simulink model "IDMF_datagenerator"  (R2022a)
settings: Solver=VariableStepAuto  StartTime=0.0  StopTime=30  FixedStep=0.05  RelTol=1e-3
PostLoadFcn:
  | %Add subfolders to path
  | addpath('virtualworld');
InitFcn:
  | startScript;
values from neighbouring files (symbols this model uses):
  angularVelocity = [0 0 -0.01]    [startScript.m]
  angularVelocityforLanding = [0 0 0]    [startScript.m]
  dronestartlocation = [-1.5 0 4]    [startScript.m]
  Dstar = -0.5    [startScript.m]
  finalHoverHeight = 2.5    [startScript.m]
  helipadLocation = [14 0.6 5]    [startScript.m]
  linearVelocity = [5 0.05 1]    [startScript.m]
  linearVelocityforHover = [0.65 0.05 0.3]    [startScript.m]
  windAVelocity = [0 0.1 0.1]    [startScript.m]
  windLVelocity = [0.1 0 0.3]    [startScript.m]
undefined symbols (not defined in the file or in its folder): fspecial, gcbh, Kanade, Lucas, Rec, SDTV, vrmfunc
libraries: visiontextngfix x11, visionconversions x9, visionanalysis x8, vrlib x7, slpidlib x3, sharedtransform x2, simulink x1
(part 1 of 3)
settings Model: Creator=91967  LastModifiedBy=sshoo
settings SolverCC: AlgebraicLoopSolver=TrustRegion
settings DebuggingCC: UnconnectedInputMsg=warning  UnconnectedOutputMsg=warning  UnconnectedLineMsg=warning  SFMachineParentedDataDiag=warning
settings SFSimCC: MATLABDynamicMemAllocThreshold=4000
settings RTWCC: DLArmComputeVersion=19.05

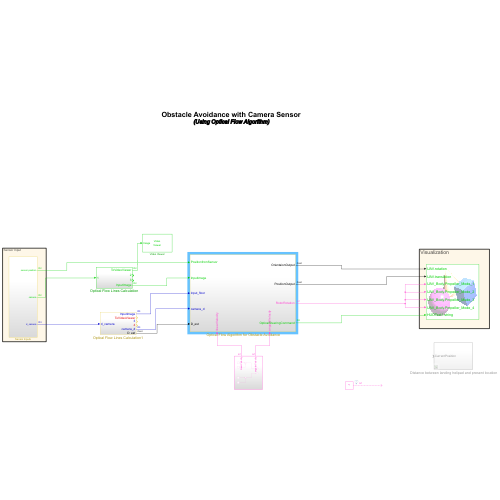
[thumbnail: Simulink's stored preview of the top-level diagram]
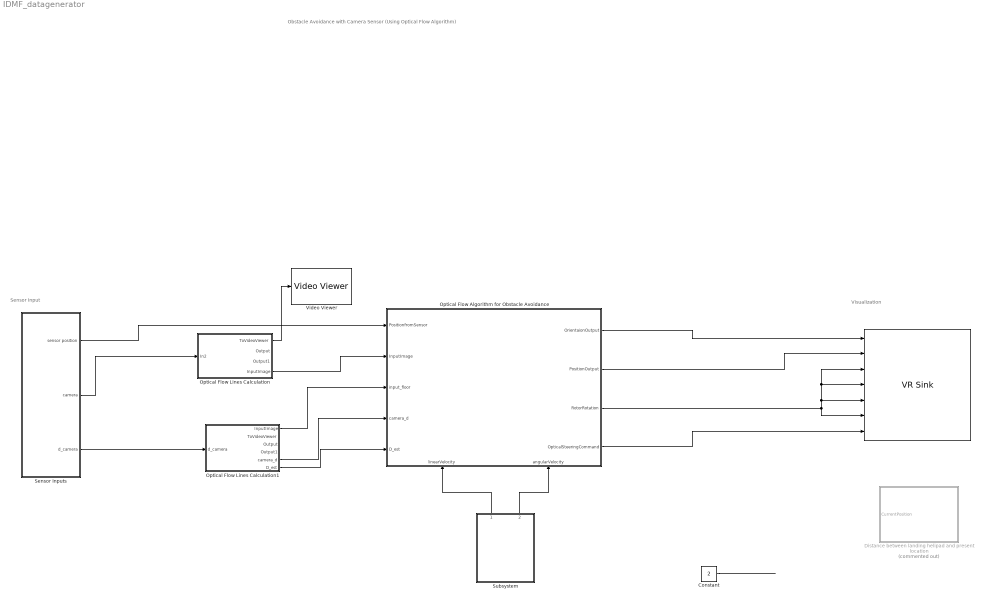
== system IDMF_datagenerator ==
  note: Sensor Input
  note: Obstacle Avoidance with Camera Sensor
      | (Using Optical Flow Algorithm)
  note: Visualization
  "    " : vrlib/VR Sink  InstantiateOnLoad=on  SampleTime=0.04  ViewEnable=on  RemoteChange=off  RemoteView=off  FieldsWritten=UAV.rotation.4.1.1.double#UAV.translation.3.1.1.double#UAV_Body.Propeller_Mode_1.1.1.1.double#UAV_Body.Propeller_Mode_2.1.1.1.double#UAV_Body.Propeller_Mode_3.1.1.1.double#UAV_Body.Propeller_Mode_4.1.1.1.double#HUDText1.string.1.-1.1.char  WorldFileName=slv3.x3d  WorldDescription=Obstacle Avoidance with Camera Sensor (Using Optical Flow Algorithm)  AutoView=off  VideoDimensions=[]  AllowVariableSize=off
  " Distance between landing helipad and present location" : Subsystem  Commented=on
  " Optical Flow Algorithm for Obstacle Avoidance" : Subsystem
      settings: PortSchema="{\"entries\":[{\"content\":{\"sides\":[{\"content\":{\"connectorIds\":[\"In1\",\"In2\",\"In3\",\"In4\",\"In5\"]},\"type\":\"ConnectorPlacement.EquallySpacedRectSide\",\"uuid\":\"626d938a-dc4f-460f-bc0f-94d4819770df\"},{\"content\":{\"connectorIds\":[\"Out1\",\"Out2\",\"Out3\",\"Out4\"],\"side\":\"RIGHT\"},\"type\":\"ConnectorPlacement.EquallySpacedRectSide\",\"uuid\":\"f8576f54-f0f3-45bb-99e7-76b9dd7ef3ed\"},{\"content\":{\"connectorIds\":[],\"side\":\"TOP\"},\"type\":\"ConnectorPlacement.EquallySpacedRectSide\",\"uuid\":\"339010c6-3d09-402d-955a-c6f9b5dbd0bd\"},{\"content\":{\"connectorIds\":[\"In6\",\"In7\"],\"side\":\"BOTTOM\"},\"type\":\"ConnectorPlacement.EquallySpacedRectSide\",\"uuid\":\"67e63212-85fa-4929-bde2-eaa65e03c106\"}]},\"type\":\"ConnectorPlacement.EquallySpacedConnector\",\"uuid\":\"635d6afa-5e1d-48cf-844f-d5ce6ee259d5\"}],\"packageUris\":[\"http://schema.mathworks.com/mf0/Connector/R2020b\"],\"version\":\"1.0\"}"
  Constant : Constant  Value=2
  Optical Flow Lines Calculation : Subsystem
  Optical Flow Lines Calculation1 : Subsystem
  Sensor Inputs : Subsystem
  Subsystem : Subsystem
  Video Viewer : VideoViewer  FigPos=[100 1042 709 500]
  wires:
  Sensor Inputs/1(sensor position) -> " Optical Flow Algorithm for Obstacle Avoidance"/1(PositionfromSensor)
  Sensor Inputs/2(camera) -> Optical Flow Lines Calculation/1(In2)
  " Optical Flow Algorithm for Obstacle Avoidance"/3(RotorRotation) -> "    "/6, "    "/4, "    "/3, "    "/5
  " Optical Flow Algorithm for Obstacle Avoidance"/4(OpticalSteeringCommand) -> "    "/7
  Sensor Inputs/3(d_camera) -> Optical Flow Lines Calculation1/1(d_camera)
  Optical Flow Lines Calculation1/1(InputImage) -> " Optical Flow Algorithm for Obstacle Avoidance"/3(input_floor)
  Optical Flow Lines Calculation/4(InputImage) -> " Optical Flow Algorithm for Obstacle Avoidance"/2(InputImage)
  Optical Flow Lines Calculation1/6(D_est) -> " Optical Flow Algorithm for Obstacle Avoidance"/5(D_est)
  Optical Flow Lines Calculation1/5(camera_d) -> " Optical Flow Algorithm for Obstacle Avoidance"/4(camera_d)
  " Optical Flow Algorithm for Obstacle Avoidance"/1(OrientaionOutput) -> "    "/1
  " Optical Flow Algorithm for Obstacle Avoidance"/2(PositionOutput) -> "    "/2
  Subsystem/1(linearVelocity) -> " Optical Flow Algorithm for Obstacle Avoidance"/6(linearVelocity)
  Subsystem/2(angularVelocity) -> " Optical Flow Algorithm for Obstacle Avoidance"/7(angularVelocity)
  Constant/1 -> ?
  Optical Flow Lines Calculation/1(ToVideoViewer) -> Video Viewer/1

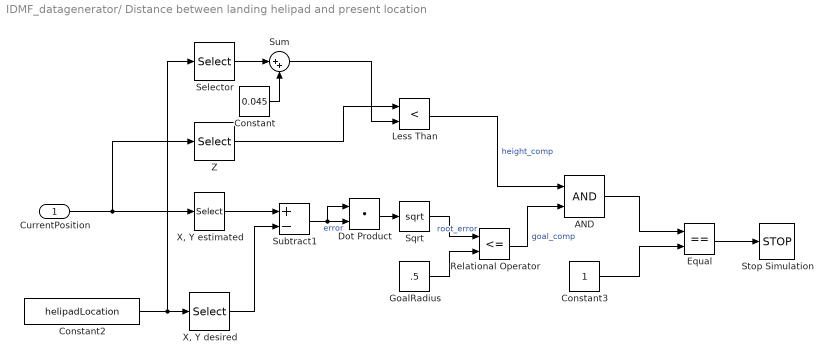
== system IDMF_datagenerator/ Distance between landing helipad and present location ==
  CurrentPosition : Inport
  AND : Logic  IconShape=distinctive  AllPortsSameDT=off  OutDataTypeStr=boolean
  Constant : Constant  Value=0.045
  Constant2 : Constant  Value=helipadLocation
  Constant3 : Constant
  Dot Product : DotProduct  OutDataTypeStr=Inherit: Inherit via internal rule
  Equal : RelationalOperator  Operator===  OutDataTypeStr=boolean  RndMeth=Simplest  InputSameDT=off
  GoalRadius : Constant  Value=.5
  Less Than : RelationalOperator  Operator=<  OutDataTypeStr=boolean  RndMeth=Simplest  InputSameDT=off
  Relational Operator : RelationalOperator  Operator=<=  OutDataTypeStr=boolean  RndMeth=Simplest  InputSameDT=off
  Selector : Selector  InputPortWidth=3  IndexOptions=Index vector (dialog)  Indices=[2]  OutputSizes=1
  Sqrt : Sqrt
  Stop Simulation : Stop
  Subtract1 : Sum  Inputs=+-
  Sum : Sum  Inputs=|++
  "X, Y desired" : Selector  InputPortWidth=3  IndexOptions=Index vector (dialog)  Indices=[1 3]  OutputSizes=1
  "X, Y estimated" : Selector  InputPortWidth=3  IndexOptions=Index vector (dialog)  Indices=[1 3]  OutputSizes=1
  Z : Selector  InputPortWidth=3  IndexOptions=Index vector (dialog)  Indices=[2]  OutputSizes=1
  wires:
  GoalRadius/1 -> Relational Operator/2
  Subtract1/1 -> Dot Product/1, Dot Product/2  "error"
  Dot Product/1 -> Sqrt/1
  Sqrt/1 -> Relational Operator/1  "root_error"
  "X, Y estimated"/1 -> Subtract1/1
  CurrentPosition/1 -> Z/1, "X, Y estimated"/1
  "X, Y desired"/1 -> Subtract1/2
  Constant3/1 -> Equal/2
  Equal/1 -> Stop Simulation/1
  Constant2/1 -> Selector/1, "X, Y desired"/1
  AND/1 -> Equal/1
  Relational Operator/1 -> AND/2  "goal_comp"
  Z/1 -> Less Than/1
  Less Than/1 -> AND/1  "height_comp"
  Selector/1 -> Sum/1
  Constant/1 -> Sum/2
  Sum/1 -> Less Than/2

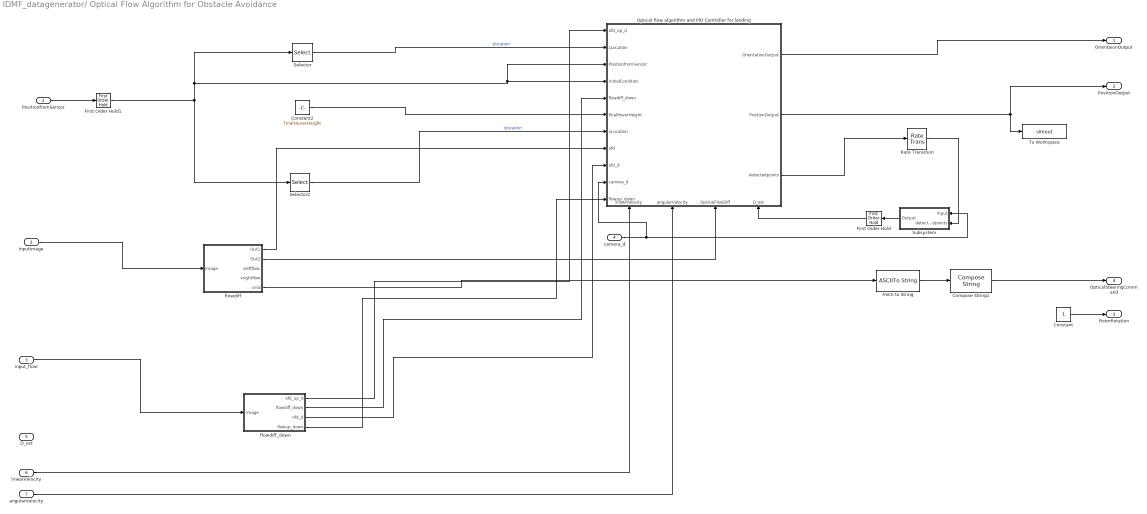
== system IDMF_datagenerator/ Optical Flow Algorithm for Obstacle Avoidance ==
  PositionfromSensor : Inport  OutDataTypeStr=double
  InputImage : Inport  Port=2
  input_floor : Inport  Port=3
  camera_d : Inport  Port=4
  D_est : Inport  Port=5
  linearVelocity : Inport  Port=6
  angularVelocity : Inport  Port=7
  ASCII to String : ASCIIToString
  Compose String1 : ComposeString  Format="\"%s\""
  Constant : Constant
  Constant2 : Constant  Value=finalHoverHeight
  First Order Hold : FirstOrderHold  ErrorTolerance=0  AllowContinuousInput=on
  First Order Hold1 : FirstOrderHold  ErrorTolerance=inf
  Optical flow algorithm and PID Controller for landing : Stateflow chart  TreatAsAtomicUnit=on
      settings: PortSchema="{\"entries\":[{\"content\":{\"sides\":[{\"content\":{\"connectorIds\":[\"In5\",\"In6\",\"In7\",\"In8\",\"In9\",\"In10\",\"In11\",\"In13\",\"In14\",\"In12\",\"In15\"]},\"type\":\"ConnectorPlacement.EquallySpacedRectSide\",\"uuid\":\"e0417acb-7520-44a1-81fe-3cf9a64aaaa4\"},{\"content\":{\"connectorIds\":[\"Out1\",\"Out2\",\"Out3\"],\"side\":\"RIGHT\"},\"type\":\"ConnectorPlacement.EquallySpacedRectSide\",\"uuid\":\"44842af9-d70e-40e5-b27b-20e9bdb5de5c\"},{\"content\":{\"connectorIds\":[],\"side\":\"TOP\"},\"type\":\"ConnectorPlacement.EquallySpacedRectSide\",\"uuid\":\"27a245c1-5cf2-418b-a56f-6add92dc71be\"},{\"content\":{\"connectorIds\":[\"In1\",\"In2\",\"In3\",\"In4\"],\"side\":\"BOTTOM\"},\"type\":\"ConnectorPlacement.EquallySpacedRectSide\",\"uuid\":\"f0be2f5a-19b7-4698-85a9-69c72a6e07e4\"}]},\"type\":\"ConnectorPlacement.EquallySpacedConnector\",\"uuid\":\"6007b39c-018d-48d6-ae79-01dba3bf1617\"}],\"packageUris\":[\"http://schema.mathworks.com/mf0/Connector/R2020b\"],\"version\":\"1.0\"}"
  Rate Transition : RateTransition  OutPortSampleTime=0.1
  Selector : Selector  InputPortWidth=3  IndexOptions=Index vector (dialog)  Indices=[2]  OutputSizes=1
  Selector2 : Selector  InputPortWidth=3  IndexOptions=Index vector (dialog)  Indices=[1]  OutputSizes=1
  Subsystem : Subsystem
  To Workspace : ToWorkspace  VariableName=simout  SaveFormat=Timeseries  SampleTime=-1
  flowdiff : Subsystem
  flowdiff_down : Subsystem
  OrientaionOutput : Outport
  PositionOutput : Outport  Port=2
  RotorRotation : Outport  Port=3
  OpticalSteeringCommand : Outport  Port=4
  wires:
  Optical flow algorithm and PID Controller for landing/2(PositionOutput) -> PositionOutput/1, To Workspace/1
  Optical flow algorithm and PID Controller for landing/1(OrientationOutput) -> OrientaionOutput/1
  ASCII to String/1 -> Compose String1/1
  Compose String1/1 -> OpticalSteeringCommand/1
  Constant/1 -> RotorRotation/1
  PositionfromSensor/1 -> First Order Hold1/1
  Selector/1 -> Optical flow algorithm and PID Controller for landing/6(zLocation)  "zlocation"
  Constant2/1 -> Optical flow algorithm and PID Controller for landing/10(finalHoverHeight)
  Selector2/1 -> Optical flow algorithm and PID Controller for landing/11(xLocation)  "xlocation"
  camera_d/1 -> Optical flow algorithm and PID Controller for landing/12(camera_d), Subsystem/1(Input)
  Optical flow algorithm and PID Controller for landing/3(detectedpoints) -> Rate Transition/1
  Rate Transition/1 -> Subsystem/2(detectedpoints)
  First Order Hold/1 -> Optical flow algorithm and PID Controller for landing/4(D_est)
  Subsystem/1(Output) -> First Order Hold/1
  input_floor/1 -> flowdiff_down/1(image)
  flowdiff_down/1(ofd_up_d) -> Optical flow algorithm and PID Controller for landing/5(ofd_up_d)
  flowdiff_down/2(flowdiff_down) -> Optical flow algorithm and PID Controller for landing/9(flowdiff_down)
  flowdiff_down/3(ofd_d) -> Optical flow algorithm and PID Controller for landing/14(ofd_d)
  flowdiff_down/4(flowup_down) -> Optical flow algorithm and PID Controller for landing/15(flowup_down)
  InputImage/1 -> flowdiff/1(image)
  flowdiff/1(Out1) -> Optical flow algorithm and PID Controller for landing/13(ofd)
  flowdiff/2(Out2) -> Optical flow algorithm and PID Controller for landing/3(OpticalFlowDiff)
  flowdiff/5(cmd) -> ASCII to String/1
  linearVelocity/1 -> Optical flow algorithm and PID Controller for landing/1(linearVelocity)
  angularVelocity/1 -> Optical flow algorithm and PID Controller for landing/2(angularVelocity)
  First Order Hold1/1 -> Selector/1, Optical flow algorithm and PID Controller for landing/7(PositionfromSensor), Optical flow algorithm and PID Controller for landing/8(InitialCondition), Selector2/1

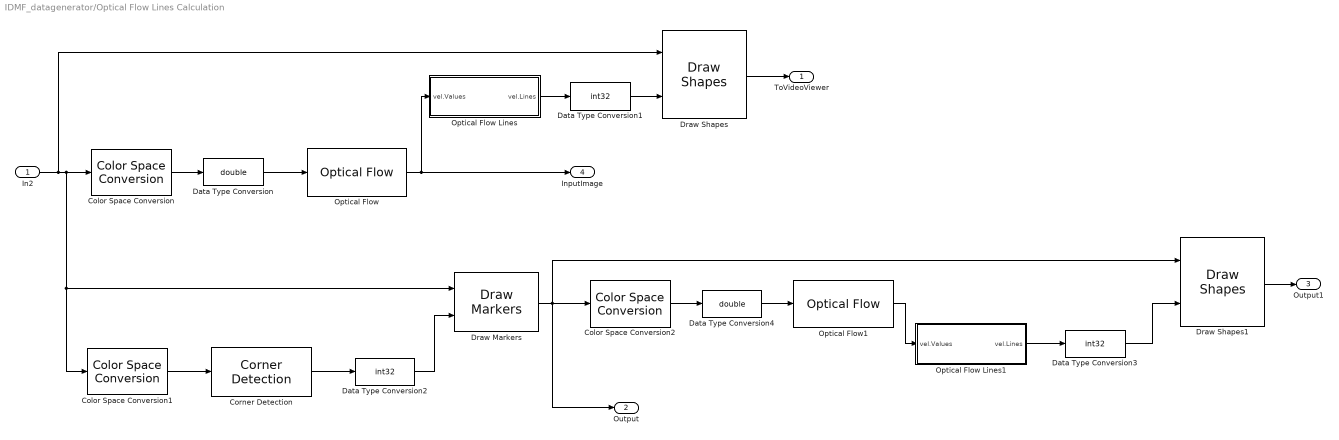
== system IDMF_datagenerator/Optical Flow Lines Calculation ==
  In2 : Inport
  Color Space Conversion : visionconversions/Color Space  Conversion  conversion=Obsolete  conversionActive=R'G'B' to intensity  wp_str=D65  rec=Rec. 601 (SDTV)  sys=1125/60/2:1  imagePorts=One multidimensional signal
  Color Space Conversion1 : visionconversions/Color Space  Conversion  conversion=Obsolete  conversionActive=R'G'B' to intensity  wp_str=D65  rec=Rec. 601 (SDTV)  sys=1125/60/2:1  imagePorts=One multidimensional signal
  Color Space Conversion2 : visionconversions/Color Space  Conversion  conversion=Obsolete  conversionActive=R'G'B' to intensity  wp_str=D65  rec=Rec. 601 (SDTV)  sys=1125/60/2:1  imagePorts=One multidimensional signal
  Corner Detection : visionanalysis/Corner Detection  method=Local intensity comparison (Rosen & Drummond)  factor=0.04  filter=fspecial('gaussian', [1 5], 1.5)  thrInten=0.1  thrAngle=112.5  output=Obsolete9b  outputInUse=Corner location  maxNum=50  thrMetric=0.005  neighborSize=[11 11]  isOutVarDim=on  roundingMode=Floor  overflowMode=off  firstCoeffMode=Specify word length  firstCoeffWordLength=16  firstCoeffFracLength=16  prodOutputMode=Binary point scaling  prodOutputWordLength=32  prodOutputFracLength=0  accumMode=Binary point scaling  accumWordLength=32  accumFracLength=0  memoryMode=Binary point scaling  memoryWordLength=32  memoryFracLength=0
      settings: SourceProductBaseCode=VP
  Data Type Conversion : DataTypeConversion  OutDataTypeStr=double  SaturateOnIntegerOverflow=off  RndMeth=Floor
  Data Type Conversion1 : DataTypeConversion  OutDataTypeStr=int32  SaturateOnIntegerOverflow=off  RndMeth=Floor
  Data Type Conversion2 : DataTypeConversion  OutDataTypeStr=int32  SaturateOnIntegerOverflow=off  RndMeth=Floor
  Data Type Conversion3 : DataTypeConversion  OutDataTypeStr=int32  SaturateOnIntegerOverflow=off  RndMeth=Floor
  Data Type Conversion4 : DataTypeConversion  OutDataTypeStr=double  SaturateOnIntegerOverflow=off  RndMeth=Floor
  Draw Markers : visiontextngfix/Draw Markers  shape=Plus  size=3  fill=off  fillClrSource=Specify via dialog  display=User-specified value  intensity=200  color=[255 0 0]  opacity=0.6  viewport=Entire image  antialiasing=off  inType=Obsolete  imagePorts=One multidimensional signal  roundingMode=Floor  overflowMode=off  memoryMode=Specify word length  memoryWordLength=16  memoryFracLength=15  prodOutputMode=Binary point scaling  prodOutputWordLength=32  prodOutputFracLength=14
      settings: SourceProductBaseCode=VP
  Draw Shapes : visiontextngfix/Draw Shapes  shape=Lines  fill=off  lineWidth=1  fillClrSource=Specify via dialog  display=User-specified value  intensity=200  color=[255 0 0]  opacity=0.6  viewport=Entire image  antialiasing=off  inType=Obsolete  imagePorts=One multidimensional signal  roundingMode=Floor  overflowMode=off  memoryMode=Specify word length  memoryWordLength=16  prodOutputMode=Binary point scaling  prodOutputWordLength=32  prodOutputFracLength=14  memoryFracLength=15
  Draw Shapes1 : visiontextngfix/Draw Shapes  shape=Lines  fill=off  lineWidth=1  fillClrSource=Specify via dialog  display=User-specified value  intensity=200  color=[255 255 0]  opacity=0.6  viewport=Entire image  antialiasing=off  inType=Obsolete  imagePorts=One multidimensional signal  roundingMode=Floor  overflowMode=off  memoryMode=Specify word length  memoryWordLength=16  prodOutputMode=Binary point scaling  prodOutputWordLength=32  prodOutputFracLength=14  memoryFracLength=15
  Optical Flow : visionanalysis/Optical Flow  method=Lucas-Kanade  gradMethod=Derivative of Gaussian  which2img=Current frame and N-th frame back  N=1  lambda=60  numInports=5  sigmaS=1.5  sigmaW=1  discardNormalFlow=off  outputCurrentImage=off  stop_criteria=When maximum number of iterations is reached  maxIter=10  maxAllowAbsDiff=eps  outVelForm=Magnitude-squared  eigTh=0.039  roundingMode=Nearest  overflowMode=on  prodOutputMode=Binary point scaling  prodOutputWordLength=32  prodOutputFracLength=20  outputMode=Binary point scaling  outputWordLength=32  outputFracLength=20
      settings: SourceProductBaseCode=VP
  Optical Flow Lines : Subsystem  mask(Optical Flow Lines){scaleFactor=1}
      mask prompts: scaleFactor "Motion vector gain:"
      mask help: Generates the coordinate points of optical flow lines.
      mask Help: Generates the coordinate points of optical flow lines. Look under its mask to see the implementation details.
  Optical Flow Lines1 : Subsystem  mask(Optical Flow Lines){scaleFactor=1}
      mask prompts: scaleFactor "Motion vector gain:"
      mask help: Generates the coordinate points of optical flow lines.
      mask Help: Generates the coordinate points of optical flow lines. Look under its mask to see the implementation details.
  Optical Flow1 : visionanalysis/Optical Flow  method=Lucas-Kanade  gradMethod=Derivative of Gaussian  which2img=Current frame and N-th frame back  N=1  lambda=1  numInports=3  sigmaS=1.5  sigmaW=1  discardNormalFlow=off  outputCurrentImage=off  stop_criteria=When maximum number of iterations is reached  maxIter=10  maxAllowAbsDiff=eps  outVelForm=Magnitude-squared  eigTh=0.0039  roundingMode=Nearest  overflowMode=on  prodOutputMode=Binary point scaling  prodOutputWordLength=32  prodOutputFracLength=20  outputMode=Binary point scaling  outputWordLength=32  outputFracLength=20
      settings: SourceProductBaseCode=VP
  ToVideoViewer : Outport
  Output : Outport  Port=2
  Output1 : Outport  Port=3
  InputImage : Outport  Port=4
  wires:
  Optical Flow Lines/1(vel.Lines) -> Data Type Conversion1/1
  Data Type Conversion1/1 -> Draw Shapes/2
  Draw Shapes/1 -> ToVideoViewer/1
  Data Type Conversion/1 -> Optical Flow/1
  Color Space Conversion/1 -> Data Type Conversion/1
  Optical Flow Lines1/1(vel.Lines) -> Data Type Conversion3/1
  Data Type Conversion3/1 -> Draw Shapes1/2
  Draw Shapes1/1 -> Output1/1
  Color Space Conversion2/1 -> Data Type Conversion4/1
  Data Type Conversion4/1 -> Optical Flow1/1
  Corner Detection/1 -> Data Type Conversion2/1
  Draw Markers/1 -> Draw Shapes1/1, Output/1, Color Space Conversion2/1
  Data Type Conversion2/1 -> Draw Markers/2
  Color Space Conversion1/1 -> Corner Detection/1
  Optical Flow1/1 -> Optical Flow Lines1/1(vel.Values)
  In2/1 -> Color Space Conversion1/1, Draw Markers/1, Color Space Conversion/1, Draw Shapes/1
  Optical Flow/1 -> Optical Flow Lines/1(vel.Values), InputImage/1

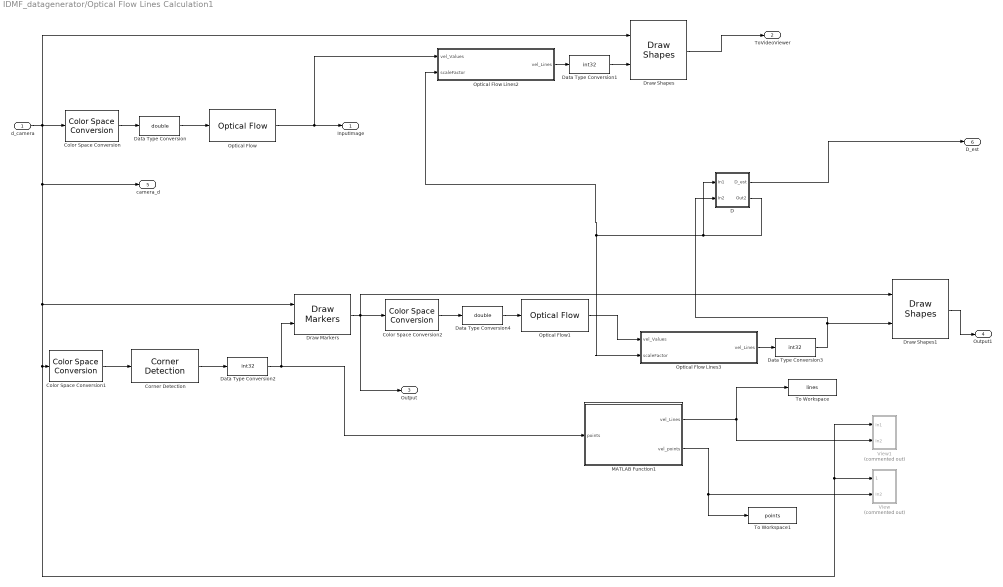
== system IDMF_datagenerator/Optical Flow Lines Calculation1 ==
  d_camera : Inport
  Color Space Conversion : visionconversions/Color Space  Conversion  conversion=Obsolete  conversionActive=R'G'B' to intensity  wp_str=D65  rec=Rec. 601 (SDTV)  sys=1125/60/2:1  imagePorts=One multidimensional signal
  Color Space Conversion1 : visionconversions/Color Space  Conversion  conversion=Obsolete  conversionActive=R'G'B' to intensity  wp_str=D65  rec=Rec. 601 (SDTV)  sys=1125/60/2:1  imagePorts=One multidimensional signal
  Color Space Conversion2 : visionconversions/Color Space  Conversion  conversion=Obsolete  conversionActive=R'G'B' to intensity  wp_str=D65  rec=Rec. 601 (SDTV)  sys=1125/60/2:1  imagePorts=One multidimensional signal
  Corner Detection : visionanalysis/Corner Detection  method=Local intensity comparison (Rosen & Drummond)  factor=0.04  filter=fspecial('gaussian', [1 5], 1.5)  thrInten=0.1  thrAngle=157.5  output=Obsolete9b  outputInUse=Corner location  maxNum=50  thrMetric=0.005  neighborSize=[15 15]  isOutVarDim=on  roundingMode=Floor  overflowMode=off  firstCoeffMode=Specify word length  firstCoeffWordLength=16  firstCoeffFracLength=16  prodOutputMode=Binary point scaling  prodOutputWordLength=32  prodOutputFracLength=0  accumMode=Binary point scaling  accumWordLength=32  accumFracLength=0  memoryMode=Binary point scaling  memoryWordLength=32  memoryFracLength=0
      settings: SourceProductBaseCode=VP
  D : Subsystem
  Data Type Conversion : DataTypeConversion  OutDataTypeStr=double  SaturateOnIntegerOverflow=off  RndMeth=Floor
  Data Type Conversion1 : DataTypeConversion  OutDataTypeStr=int32  SaturateOnIntegerOverflow=off  RndMeth=Floor
  Data Type Conversion2 : DataTypeConversion  OutDataTypeStr=int32  SaturateOnIntegerOverflow=off  RndMeth=Floor
  Data Type Conversion3 : DataTypeConversion  OutDataTypeStr=int32  SaturateOnIntegerOverflow=off  RndMeth=Floor
  Data Type Conversion4 : DataTypeConversion  OutDataTypeStr=double  SaturateOnIntegerOverflow=off  RndMeth=Floor
  Draw Markers : visiontextngfix/Draw Markers  shape=Plus  size=3  fill=off  fillClrSource=Specify via dialog  display=User-specified value  intensity=200  color=[255 0 0]  opacity=0.6  viewport=Entire image  antialiasing=off  inType=Obsolete  imagePorts=One multidimensional signal  roundingMode=Floor  overflowMode=off  memoryMode=Specify word length  memoryWordLength=16  memoryFracLength=15  prodOutputMode=Binary point scaling  prodOutputWordLength=32  prodOutputFracLength=14
      settings: SourceProductBaseCode=VP
  Draw Shapes : visiontextngfix/Draw Shapes  shape=Lines  fill=off  lineWidth=1  fillClrSource=Specify via dialog  display=User-specified value  intensity=200  color=[255 255 0]  opacity=0.6  viewport=Entire image  antialiasing=off  inType=Obsolete  imagePorts=One multidimensional signal  roundingMode=Floor  overflowMode=off  memoryMode=Specify word length  memoryWordLength=16  prodOutputMode=Binary point scaling  prodOutputWordLength=32  prodOutputFracLength=14  memoryFracLength=15
  Draw Shapes1 : visiontextngfix/Draw Shapes  shape=Lines  fill=off  lineWidth=1  fillClrSource=Specify via dialog  display=User-specified value  intensity=200  color=[255 255 0]  opacity=0.6  viewport=Entire image  antialiasing=off  inType=Obsolete  imagePorts=One multidimensional signal  roundingMode=Floor  overflowMode=off  memoryMode=Specify word length  memoryWordLength=16  prodOutputMode=Binary point scaling  prodOutputWordLength=32  prodOutputFracLength=14  memoryFracLength=15
  MATLAB Function1 : MATLAB Function  TreatAsAtomicUnit=on
  Optical Flow : visionanalysis/Optical Flow  method=Lucas-Kanade  gradMethod=Derivative of Gaussian  which2img=Current frame and N-th frame back  N=1  lambda=1  numInports=9  sigmaS=1.5  sigmaW=1  discardNormalFlow=off  outputCurrentImage=off  stop_criteria=When maximum number of iterations is reached  maxIter=10  maxAllowAbsDiff=eps  outVelForm=Magnitude-squared  eigTh=0.039  roundingMode=Nearest  overflowMode=on  prodOutputMode=Binary point scaling  prodOutputWordLength=32  prodOutputFracLength=20  outputMode=Binary point scaling  outputWordLength=32  outputFracLength=20
      settings: SourceProductBaseCode=VP
  Optical Flow Lines2 : MATLAB Function  TreatAsAtomicUnit=on
  Optical Flow Lines3 : MATLAB Function  TreatAsAtomicUnit=on
  Optical Flow1 : visionanalysis/Optical Flow  method=Lucas-Kanade  gradMethod=Derivative of Gaussian  which2img=Current frame and N-th frame back  N=1  lambda=1  numInports=9  sigmaS=3  sigmaW=1  discardNormalFlow=off  outputCurrentImage=off  stop_criteria=When maximum number of iterations is reached  maxIter=10  maxAllowAbsDiff=eps  outVelForm=Horizontal and vertical components in complex form  eigTh=2  roundingMode=Nearest  overflowMode=on  prodOutputMode=Binary point scaling  prodOutputWordLength=32  prodOutputFracLength=20  outputMode=Binary point scaling  outputWordLength=32  outputFracLength=20
      settings: SourceProductBaseCode=VP
  To Workspace : ToWorkspace  VariableName=lines  SaveFormat=Timeseries  SampleTime=-1
  To Workspace1 : ToWorkspace  VariableName=points  SaveFormat=Timeseries  SampleTime=-1
  View : Subsystem  Commented=on
  View1 : Subsystem  Commented=on
  InputImage : Outport
  ToVideoViewer : Outport  Port=2
  Output : Outport  Port=3
  Output1 : Outport  Port=4
  camera_d : Outport  Port=5
  D_est : Outport  Port=6
  wires:
  Optical Flow/1 -> Optical Flow Lines2/1(vel_Values), InputImage/1
  Color Space Conversion/1 -> Data Type Conversion/1
  Data Type Conversion/1 -> Optical Flow/1
  Draw Markers/1 -> Output/1, Draw Shapes1/1, Color Space Conversion2/1
  Color Space Conversion1/1 -> Corner Detection/1
  Data Type Conversion2/1 -> MATLAB Function1/1(points), Draw Markers/2
  Corner Detection/1 -> Data Type Conversion2/1
  Draw Shapes/1 -> ToVideoViewer/1
  Optical Flow1/1 -> Optical Flow Lines3/1(vel_Values)
  Optical Flow Lines3/1(vel_Lines) -> Data Type Conversion3/1
  Data Type Conversion3/1 -> D/2(In2), Draw Shapes1/2
  Draw Shapes1/1 -> Output1/1
  Data Type Conversion4/1 -> Optical Flow1/1
  Color Space Conversion2/1 -> Data Type Conversion4/1
  Data Type Conversion1/1 -> Draw Shapes/2
  Optical Flow Lines2/1(vel_Lines) -> Data Type Conversion1/1
  d_camera/1 -> View1/1(In1), View/1(d_camera), Color Space Conversion1/1, Draw Markers/1, camera_d/1, Draw Shapes/1, Color Space Conversion/1
  MATLAB Function1/2(vel_points) -> To Workspace1/1, View/2(In2)
  D/2(Out2) -> Optical Flow Lines2/2(scaleFactor), Optical Flow Lines3/2(scaleFactor), D/1(In1)
  D/1(D_est) -> D_est/1
  MATLAB Function1/1(vel_Lines) -> View1/2(In2), To Workspace/1

== system IDMF_datagenerator/Sensor Inputs ==
  note: Do not change the Quadcopter Camera View in the On-board Camera and Virtual Reality Sensors block. This will affect the Optical Flow algorithm since we need the images from the front camera.
  On-Board Camera : S-Function  InstantiateOnLoad=on  LoadFcn=vrmfunc('FnLoad', gcbh);  InitFcn=""  StartFcn=vrmfunc('FnSimStatus', gcbh, 'running')  StopFcn=vrmfunc('FnStop', gcbh)  FunctionName=vrsfunc  Parameters=SampleTime, VideoDimensions, false  SFunctionDeploymentMode=off  EnableBusSupport=off  mask(Virtual Reality Sink){SampleTime=0.04, ViewEnable=on, RemoteChange=off, RemoteView=off, FieldsWritten=, WorldFileName=slv3.x3d, WorldDescription=Obstacle avoidance using  Optical Flow Algorithm for UAV, AutoView=off, VideoDimensions=[320 480], AllowVariableSize=off, FigureProperties={'Position', 'Name', 'Viewpoint', 'CameraBound', 'CameraDirection', 'CameraPosition', 'CameraUpVector', 'ZoomFactor', 'Antialiasing', 'Headlight', 'Lighting', 'NavPanel', 'Sound', 'StatusBar', 'Stereo3D', 'Stereo3DCameraOffset', 'Stereo3DHIT', 'ToolBar', 'Textures', 'Transparency', 'Triad', 'Wireframe', 'NavZones', 'NavMode', 'NavSpeed', 'CaptureFileFormat', 'CaptureFileName', 'Record2DCompressMethod', 'Record2DCompressQuality', 'Record2D', 'Record2DFileName', 'Record2DFPS'; [5.8600000000000000e+02   6.0000000000000000e+01   4.8000000000000000e+02   3.2000000000000000e+02], 'UAV Competition Scene', 'Bird''s Eye', 'on', [0.0000000000000000e+00   0.0000000000000000e+00  -1.0000000000000000e+00], [0.0000000000000000e+00   0.0000000000000000e+00   0.0000000000000000e+00], [0.0000000000000000e+00   1.0000000000000000e+00   0.0000000000000000e+00], [1.0000000000000000e+00], 'on', 'on', 'on', 'none', 'on', 'off', 'off', [1.0000000149011612e-01], [0.0000000000000000e+00], 'off', 'on', 'on', 'none', 'off', 'off', 'fly', 'normal', 'tif', '%f_anim_%n.tif', 'auto', [7.5000000000000000e+01], 'off', '***video***', 'auto'}}
      mask prompts: SampleTime "Sample Time"; ViewEnable "View"; RemoteChange "Remote Change"; RemoteView "Remote View"; FieldsWritten "Fields Written"; WorldFileName "World File Name"; WorldDescription "World Description"; VideoDimensions "Video Dimensions"; AllowVariableSize "Allow Variable Size"; FigureProperties "Figure Properties"
      mask help: Controls the selected fields of a virtual world according to given inputs.
      mask init:
      | set_param(gcbh, 'MaskDisplay', vrmfunc('FnIcon'));
      settings: CopyFcn=vrmfunc('FnCopy', gcbh);  DeleteFcn=vrmfunc('FnDelete', gcbh);  PreSaveFcn=vrmfunc('FnPreSave', gcbh);  PauseFcn=vrmfunc('FnSimStatus', gcbh, 'paused');  ContinueFcn=vrmfunc('FnSimStatus', gcbh, 'running');  DestroyFcn=vrmfunc('FnDestroy', gcbh);  OpenFcn=vrmfunc('FnOpen', gcbh);  CloseFcn=vrmfunc('FnClose', gcbh);
      mask Help: helpview(vrmfunc('FnHelpTopic'), 'vr_vrtovideo');
      mask Display: image(imread('vrblockicon.png'));
  VR To Video : vrlib/VR To Video  InstantiateOnLoad=on  SampleTime=0.1  ViewEnable=on  RemoteChange=off  RemoteView=off  WorldFileName=virtualworld\slv3.x3d  WorldDescription=Obstacle Avoidance with Camera Sensor (Using Optical Flow Algorithm)  AutoView=off  VideoDimensions=[320 480]  AllowVariableSize=off  FigureProperties="{'Position', 'Name', 'Viewpoint', 'CameraBound', 'CameraDirection', 'CameraPosition', 'CameraUpVector', 'ZoomFactor', 'Antialiasing', 'Headlight', 'Lighting', 'NavPanel', 'Sound', 'StatusBar', 'Stereo3D', 'Stereo3DCameraOffset', 'Stereo3DHIT', 'ToolBar', 'Textures', 'Transparency', 'Triad', 'Wireframe', 'NavZones', 'NavMode', 'NavSpeed', 'CaptureFileFormat', 'CaptureFileName', 'Record2DCompressMethod', 'Record2DCompressQuality', 'Record2D', 'Record2DFileName', 'Record2DFPS'; [5.0000000000000000e+00   6.0000000000000000e+01   4.8000000000000000e+02   3.2000000000000000e+02], 'Obstacle Avoidance with Camera Sensor (Using Optical Flow Algorithm)', 'UAV Camera Looking Down', 'on', [0.0000000000000000e+00   0.0000000000000000e+00  -1.0000000000000000e+00], [0.0000000000000000e+00   0.0000000000000000e+00   0.0000000000000000e+00], [0.0000000000000000e+00   1.0000000000000000e+00   0.0000000000000000e+00], [1.0000000000000000e+00], 'on', 'on', 'on', 'none', 'on', 'off', 'off', [1.0000000149011612e-01], [0.0000000000000000e+00], 'off', 'on', 'on', 'none', 'off', 'off', 'fly', 'normal', 'tif', '%f_anim_%n.tif', 'auto', [7.5000000000000000e+01], 'off', '***video***', 'auto'}"
      settings: SourceProductBaseCode=SL
  Virtual Reality Sensors : vrlib/VR Source  InstantiateOnLoad=on  SampleTime=0.04  ViewEnable=on  RemoteChange=off  RemoteView=off  FieldsRead=UAV.translation.1.3.1.double  WorldFileName=slv3.x3d  WorldDescription=UAV Competition Scene  AutoView=on  VideoDimensions=[]  AllowVariableSize=off  FigureProperties="{'Position', 'Name', 'Viewpoint', 'CameraBound', 'CameraDirection', 'CameraPosition', 'CameraUpVector', 'ZoomFactor', 'Antialiasing', 'Headlight', 'Lighting', 'NavPanel', 'Sound', 'StatusBar', 'Stereo3D', 'Stereo3DCameraOffset', 'Stereo3DHIT', 'ToolBar', 'Textures', 'Transparency', 'Triad', 'Wireframe', 'NavZones', 'NavMode', 'NavSpeed', 'CaptureFileFormat', 'CaptureFileName', 'Record2DCompressMethod', 'Record2DCompressQuality', 'Record2D', 'Record2DFileName', 'Record2DFPS'; [1.7500000000000000e+02   1.3400000000000000e+02   9.2300000000000000e+02   7.1700000000000000e+02], 'Obstacle Avoidance with Camera Sensor (Using Optical Flow Algorithm)', 'Ride on the UAV Tail', 'on', [0.0000000000000000e+00   0.0000000000000000e+00  -1.0000000000000000e+00], [0.0000000000000000e+00   0.0000000000000000e+00   0.0000000000000000e+00], [0.0000000000000000e+00   1.0000000000000000e+00   0.0000000000000000e+00], [1.0000000000000000e+00], 'off', 'on', 'on', 'halfbar', 'on', 'on', 'off', [1.0000000149011612e-01], [0.0000000000000000e+00], 'on', 'on', 'on', 'none', 'off', 'off', 'fly', 'normal', 'tif', '%f_anim_%n.tif', 'auto', [7.5000000000000000e+01], 'off', '%f_anim_%n.avi', 'auto'}"
      settings: SourceProductBaseCode=SL
  sensor position : Outport
  camera : Outport  Port=2
  d_camera : Outport  Port=3
  wires:
  On-Board Camera/1 -> camera/1
  Virtual Reality Sensors/1 -> sensor position/1
  VR To Video/1 -> d_camera/1

== system IDMF_datagenerator/Subsystem ==
  Constant : Constant  Value=windAVelocity
  Constant1 : Constant  Value=angularVelocityforLanding
  Constant2 : Constant  Value=windLVelocity
  Constant3 : Constant  Value=linearVelocityforHover
  Sum : Sum  Inputs=|++
  Sum1 : Sum  Inputs=|++
  linearVelocity : Outport
  angularVelocity : Outport  Port=2
  wires:
  Constant3/1 -> Sum/1
  Sum/1 -> linearVelocity/1
  Constant2/1 -> Sum/2
  Sum1/1 -> angularVelocity/1
  Constant1/1 -> Sum1/2
  Constant/1 -> Sum1/1

== system IDMF_datagenerator/ Optical Flow Algorithm for Obstacle Avoidance/Optical flow algorithm and PID Controller for landing/ControlAlgorithm_ ==
  note: distance without known location
      | movement of landing
      | multi marker
      | gpu acuuracy modelled
  note: Hover to the given height first as mentioned by finalHoverHeight.
  PositionfromSensor : Inport
  Action Port : ActionPort
      settings: CopyFcn=Stateflow.SLINSF.SimulinkMan.removeBlockPreDeleteFcn  PreDeleteFcn=Stateflow.SLINSF.SimulinkMan.unsafePredeleteFcn
  Bus Creator1 : BusCreator  Inputs=3
  Integrator1 : Integrator  InitialConditionSource=external  UpperSaturationLimit=0.5  LowerSaturationLimit=-0.5  ZeroCross=off
  Integrator2 : Integrator  Commented=on  InitialConditionSource=external  LimitOutput=on  UpperSaturationLimit=[40 10 20]  LowerSaturationLimit=[-5 0 -5]  ZeroCross=off
  Reference2 : Constant  Value=helipadLocation(2)
  Saturation : Saturate
  Selector2 : Selector  InputPortWidth=3  IndexOptions=Index vector (dialog)  Indices=[2]  OutputSizes=1
  Selector3 : Selector  InputPortWidth=3  IndexOptions=Index vector (dialog)  Indices=[3]  OutputSizes=1
  Selector4 : Selector  InputPortWidth=3  IndexOptions=Index vector (dialog)  Indices=[1]  OutputSizes=1
  Sum2 : Sum  Inputs=+-|
  PositionOutput : Outport
  wires:
  Sum2/1 -> Saturation/1
  Reference2/1 -> Sum2/1
  Bus Creator1/1 -> PositionOutput/1
  Selector3/1 -> Bus Creator1/3
  Selector2/1 -> Integrator1/2, Sum2/2
  Selector4/1 -> Bus Creator1/1
  PositionfromSensor/1 -> Integrator2/2, Selector3/1, Selector4/1, Selector2/1
  Saturation/1 -> Integrator1/1
  Integrator1/1 -> Bus Creator1/2

== system IDMF_datagenerator/ Optical Flow Algorithm for Obstacle Avoidance/Optical flow algorithm and PID Controller for landing/DroneLanding ==
  PositionfromSensor : Inport
  Action Port : ActionPort
      settings: CopyFcn=Stateflow.SLINSF.SimulinkMan.removeBlockPreDeleteFcn  PreDeleteFcn=Stateflow.SLINSF.SimulinkMan.unsafePredeleteFcn
  Bus Creator1 : BusCreator  Inputs=3
  Integrator1 : Integrator  InitialConditionSource=external  LimitOutput=on  UpperSaturationLimit=5  LowerSaturationLimit=-5  ZeroCross=off
  Reference2 : Constant  Value=helipadLocation(2)
  Saturation : Saturate
  Selector2 : Selector  InputPortWidth=3  IndexOptions=Index vector (dialog)  Indices=[2]  OutputSizes=1
  Selector3 : Selector  InputPortWidth=3  IndexOptions=Index vector (dialog)  Indices=[3]  OutputSizes=1
  Selector4 : Selector  InputPortWidth=3  IndexOptions=Index vector (dialog)  Indices=[1]  OutputSizes=1
  Sum2 : Sum  Inputs=+-|
  PositionOutput : Outport
  wires:
  Integrator1/1 -> Bus Creator1/2
  Saturation/1 -> Integrator1/1
  Bus Creator1/1 -> PositionOutput/1
  Selector2/1 -> Integrator1/2, Sum2/2
  Selector3/1 -> Bus Creator1/3
  PositionfromSensor/1 -> Selector3/1, Selector4/1, Selector2/1
  Reference2/1 -> Sum2/1
  Selector4/1 -> Bus Creator1/1
  Sum2/1 -> Saturation/1

== system IDMF_datagenerator/ Optical Flow Algorithm for Obstacle Avoidance/Optical flow algorithm and PID Controller for landing/DroneLanding1 ==
  PositionfromSensor : Inport
  Action Port : ActionPort
      settings: CopyFcn=Stateflow.SLINSF.SimulinkMan.removeBlockPreDeleteFcn  PreDeleteFcn=Stateflow.SLINSF.SimulinkMan.unsafePredeleteFcn
  Bus Creator1 : BusCreator  Inputs=3
  Integrator1 : Integrator  InitialConditionSource=external  LimitOutput=on  UpperSaturationLimit=5  LowerSaturationLimit=-5  ZeroCross=off
  Reference2 : Constant  Value=helipadLocation(2)
  Saturation : Saturate
  Selector2 : Selector  InputPortWidth=3  IndexOptions=Index vector (dialog)  Indices=[2]  OutputSizes=1
  Selector3 : Selector  InputPortWidth=3  IndexOptions=Index vector (dialog)  Indices=[3]  OutputSizes=1
  Selector4 : Selector  InputPortWidth=3  IndexOptions=Index vector (dialog)  Indices=[1]  OutputSizes=1
  Sum2 : Sum  Inputs=+-|
  PositionOutput : Outport
  wires:
  Integrator1/1 -> Bus Creator1/2
  Saturation/1 -> Integrator1/1
  Bus Creator1/1 -> PositionOutput/1
  Selector2/1 -> Integrator1/2, Sum2/2
  Selector3/1 -> Bus Creator1/3
  PositionfromSensor/1 -> Selector3/1, Selector4/1, Selector2/1
  Reference2/1 -> Sum2/1
  Selector4/1 -> Bus Creator1/1
  Sum2/1 -> Saturation/1

== system IDMF_datagenerator/ Optical Flow Algorithm for Obstacle Avoidance/Optical flow algorithm and PID Controller for landing/DroneLanding2 ==
  PositionfromSensor : Inport
  Action Port : ActionPort
      settings: CopyFcn=Stateflow.SLINSF.SimulinkMan.removeBlockPreDeleteFcn  PreDeleteFcn=Stateflow.SLINSF.SimulinkMan.unsafePredeleteFcn
  Bus Creator1 : BusCreator  Inputs=3
  Integrator1 : Integrator  InitialConditionSource=external  LimitOutput=on  UpperSaturationLimit=5  LowerSaturationLimit=-5  ZeroCross=off
  Reference2 : Constant  Value=helipadLocation(2)
  Saturation : Saturate
  Selector2 : Selector  InputPortWidth=3  IndexOptions=Index vector (dialog)  Indices=[2]  OutputSizes=1
  Selector3 : Selector  InputPortWidth=3  IndexOptions=Index vector (dialog)  Indices=[3]  OutputSizes=1
  Selector4 : Selector  InputPortWidth=3  IndexOptions=Index vector (dialog)  Indices=[1]  OutputSizes=1
  Sum2 : Sum  Inputs=+-|
  PositionOutput : Outport
  wires:
  Integrator1/1 -> Bus Creator1/2
  Saturation/1 -> Integrator1/1
  Bus Creator1/1 -> PositionOutput/1
  Selector2/1 -> Integrator1/2, Sum2/2
  Selector3/1 -> Bus Creator1/3
  PositionfromSensor/1 -> Selector3/1, Selector4/1, Selector2/1
  Reference2/1 -> Sum2/1
  Selector4/1 -> Bus Creator1/1
  Sum2/1 -> Saturation/1

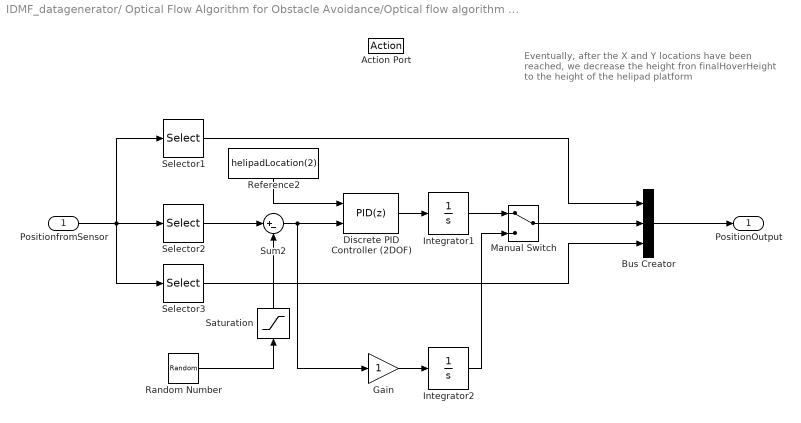
== system IDMF_datagenerator/ Optical Flow Algorithm for Obstacle Avoidance/Optical flow algorithm and PID Controller for landing/DroneLanding_ ==
  note: Eventually, after the X and Y locations have been reached, we decrease the height fron finalHoverHeight to the height of the helipad platform
  PositionfromSensor : Inport
  Action Port : ActionPort
      settings: CopyFcn=Stateflow.SLINSF.SimulinkMan.removeBlockPreDeleteFcn  PreDeleteFcn=Stateflow.SLINSF.SimulinkMan.unsafePredeleteFcn
  Bus Creator : BusCreator  Inputs=3
  Discrete PID Controller (2DOF) : slpidlib/PID Controller (2DOF)  Controller=PID  Form=Parallel  TimeDomain=Discrete-time  UseExternalTs=off  SampleTime=-1  IntegratorMethod=Forward Euler  FilterMethod=Forward Euler  ControllerParametersSource=internal  P=1.5  I=1  UseKiTs=off  D=0.5  N=1  UseFilter=on  b=1  c=1  TunerSelectOption=Transfer Function Based (PID Tuner App)  InitialConditionSource=internal  InitialConditionForIntegrator=finalHoverHeight  InitialConditionForFilter=0  DifferentiatorICPrevScaledInput=0  ExternalReset=none  TrackingMode=off  Kt=1  LimitOutput=on  SatLimitsSource=internal  UpperSaturationLimit=1  LowerSaturationLimit=-1  LinearizeAsGain=off  AntiWindupMode=none  Kb=1  POutMin=[]  POutMax=[]  IOutMin=[]  IOutMax=[]  DOutMin=[]  DOutMax=[]  NOutMin=[]  NOutMax=[]  bOutMin=[]  bOutMax=[]  cOutMin=[]  cOutMax=[]  SumOutMin=[]  SumOutMax=[]  SaturationOutMin=[]  SaturationOutMax=[]  PParamMin=[]  PParamMax=[]  IParamMin=[]  IParamMax=[]  DParamMin=[]  DParamMax=[]  NParamMin=[]  NParamMax=[]  bParamMin=[]  bParamMax=[]  cParamMin=[]  cParamMax=[]  KbParamMin=[]  KbParamMax=[]  KtParamMin=[]  KtParamMax=[]  KbOutMin=[]  KbOutMax=[]  KtOutMin=[]  KtOutMax=[]  IntegratorOutMin=[]  IntegratorOutMax=[]  FilterOutMin=[]  FilterOutMax=[]  SumI1OutMin=[]  SumI1OutMax=[]  SumI2OutMin=[]  SumI2OutMax=[]  SumI3OutMin=[]  SumI3OutMax=[]  SumI4OutMin=[]  SumI4OutMax=[]  SumDOutMin=[]  SumDOutMax=[]  Sum1OutMin=[]  Sum1OutMax=[]  Sum2OutMin=[]  Sum2OutMax=[]  Sum3OutMin=[]  Sum3OutMax=[]  DifferentiatorOutMin=[]  DifferentiatorOutMax=[]  FilterDiffOutCoefMin=[]  FilterDiffOutCoefMax=[]  ReciprocalOutMin=[]  ReciprocalOutMax=[]  SumDenOutMin=[]  SumDenOutMax=[]  SumNumOutMin=[]  SumNumOutMax=[]  DivideOutMin=[]  DivideOutMax=[]  UdiffTsProdOutMin=[]  UdiffTsProdOutMax=[]  NTsProdOutMin=[]  NTsProdOutMax=[]  UintegralTsProdOutMin=[]  UintegralTsProdOutMax=[]  UngainTsProdOutMin=[]  UngainTsProdOutMax=[]  IntegratorContinuousStateAttributes=''  IntegratorStateMustResolveToSignalObject=off  IntegratorRTWStateStorageClass=Auto  FilterContinuousStateAttributes=''  FilterStateMustResolveToSignalObject=off  FilterRTWStateStorageClass=Auto  ParallelPVariant=InternalParameters  IdealPVariant=Disabled  IVariant=InternalParameters  DVariant=InternalParameters  bVariant=InternalParameters  cVariant=InternalParameters  IntegratorVariant=Discrete  SatVariant=Enabled  AWVariant=Passthrough  PCopyVariant=Disabled  TRVariant=Disabled  FdbkBlocksVariant=Forward  IdealPFdbkVariant=Disabled  SatFdbkVariant=Disabled  DerivativeFilterVariant=ForwardEulerFilter  NVariant=InternalParameters  NCopyVariant=Disabled  FilterICVariant=InternalICsFilter  IntegratorICVariant=InternalICs  ExternalResetVariant=Disabled  TRSumVariant=Passthrough  SumFdbkVariant=Disabled  SumVariant=Sum_PID  TsampFilterVariant=InternalTs  TsampNgainVariant=Passthrough  TsampIntegralVariant=Passthrough  ExternalSaturationOutDataTypeStr=Inherit: Same as second input
      settings: SourceProductBaseCode=SL
  Gain : Gain
  Integrator1 : Integrator  InitialCondition=finalHoverHeight  UpperSaturationLimit=[40 10 20]  LowerSaturationLimit=[-5 0 -5]  ZeroCross=off
  Integrator2 : Integrator  InitialCondition=finalHoverHeight  UpperSaturationLimit=[40 10 20]  LowerSaturationLimit=[-5 0 -5]  ZeroCross=off
  Manual Switch : ManualSwitch
  Random Number : RandomNumber  SampleTime=0
  Reference2 : Constant  Value=helipadLocation(2)
  Saturation : Saturate  UpperLimit=0.1  LowerLimit=-0.1
  Selector1 : Selector  InputPortWidth=3  IndexOptions=Index vector (dialog)  Indices=[1]  OutputSizes=1
  Selector2 : Selector  InputPortWidth=3  IndexOptions=Index vector (dialog)  Indices=[2]  OutputSizes=1
  Selector3 : Selector  InputPortWidth=3  IndexOptions=Index vector (dialog)  Indices=[3]  OutputSizes=1
  Sum2 : Sum  Inputs=|+-
  PositionOutput : Outport
  wires:
  PositionfromSensor/1 -> Selector3/1, Selector1/1, Selector2/1
  Reference2/1 -> Discrete PID Controller (2DOF)/1
  Sum2/1 -> Discrete PID Controller (2DOF)/2, Gain/1
  Selector1/1 -> Bus Creator/1
  Selector3/1 -> Bus Creator/3
  Bus Creator/1 -> PositionOutput/1
  Random Number/1 -> Saturation/1
  Saturation/1 -> Sum2/2
  Selector2/1 -> Sum2/1
  Gain/1 -> Integrator2/1
  Integrator2/1 -> Manual Switch/2
  Manual Switch/1 -> Bus Creator/2
  Discrete PID Controller (2DOF)/1 -> Integrator1/1
  Integrator1/1 -> Manual Switch/1

== system IDMF_datagenerator/ Optical Flow Algorithm for Obstacle Avoidance/Optical flow algorithm and PID Controller for landing/DroneOrientationEstimation.ControlAlgorithm_ ==
  Action Port : ActionPort
      settings: CopyFcn=Stateflow.SLINSF.SimulinkMan.removeBlockPreDeleteFcn  PreDeleteFcn=Stateflow.SLINSF.SimulinkMan.unsafePredeleteFcn
  Constant : Constant  Value=angularVelocityforLanding
  Gain2 : Gain  Gain=[-1 1 1 1]
  Integrator1 : Integrator
  Rotation Angles to Direction Cosine Matrix : sharedtransform/Rotation Angles to Direction Cosine Matrix  rotationOrder=YZX  aMode=aMode
      settings: SourceProductBaseCode=AE,PW,DR,MT,VE
  Rotation Matrix to VRML Rotation1 : vrlib/Utilities/Rotation Matrix to VR Rotation  maxzero=1e-12
      settings: SourceProductBaseCode=SL
  Transpose : Math  Operator=transpose
  VR Signal Expander2 : vrlib/VR Signal Expander  outwidth=4  outidx=[1 2 3 4]
  OrientationOutput : Outport
  wires:
  Rotation Matrix to VRML Rotation1/1 -> Gain2/1
  Constant/1 -> Integrator1/1
  Rotation Angles to Direction Cosine Matrix/1 -> Transpose/1
  Transpose/1 -> Rotation Matrix to VRML Rotation1/1
  VR Signal Expander2/1 -> OrientationOutput/1
  Integrator1/1 -> Rotation Angles to Direction Cosine Matrix/1
  Gain2/1 -> VR Signal Expander2/1

== system IDMF_datagenerator/ Optical Flow Algorithm for Obstacle Avoidance/Optical flow algorithm and PID Controller for landing/DroneOrientationEstimation.OpticalFlowAlgorithm_ ==
  note: If the output from the Sign block is Positive, drone should move away
      | from the left side, i.e. Clockwise Rotation. Also, if the output from the Sign
      |  block is Negative, drone will move away from the right side..ie,
      | Anticlockwise Rotation.
  note: Steering Angular Velocities
  OpticalFlowDiff : Inport
  Action Port : ActionPort
      settings: CopyFcn=Stateflow.SLINSF.SimulinkMan.removeBlockPreDeleteFcn  PreDeleteFcn=Stateflow.SLINSF.SimulinkMan.unsafePredeleteFcn
  Constant2 : Constant  Value=angularVelocity
  Gain1 : Gain  Gain=-1
  Gain2 : Gain  Gain=[-1 1 1 1]
  Integrator1 : Integrator
  Rotation Angles to Direction Cosine Matrix : sharedtransform/Rotation Angles to Direction Cosine Matrix  rotationOrder=YZX  aMode=aMode
      settings: SourceProductBaseCode=AE,PW,DR,MT,VE
  Rotation Matrix to VRML Rotation1 : vrlib/Utilities/Rotation Matrix to VR Rotation  maxzero=1e-12
      settings: SourceProductBaseCode=SL
  Sign : Signum
  Switch : Switch  Criteria=u2 > Threshold  SaturateOnIntegerOverflow=off  InputSameDT=off
  Transpose : Math  Operator=transpose
  VR Signal Expander2 : vrlib/VR Signal Expander  outwidth=4  outidx=[1 2 3 4]
  OrientationOutput : Outport
  wires:
  Transpose/1 -> Rotation Matrix to VRML Rotation1/1
  Integrator1/1 -> Rotation Angles to Direction Cosine Matrix/1
  VR Signal Expander2/1 -> OrientationOutput/1
  OpticalFlowDiff/1 -> Sign/1
  Rotation Angles to Direction Cosine Matrix/1 -> Transpose/1
  Rotation Matrix to VRML Rotation1/1 -> Gain2/1
  Switch/1 -> Integrator1/1
  Gain2/1 -> VR Signal Expander2/1
  Constant2/1 -> Switch/3, Gain1/1  "[W_X W_Z -1*W_Y]"
  Gain1/1 -> Switch/1  "[W_X W_Z -1*W_Y]"
  Sign/1 -> Switch/2

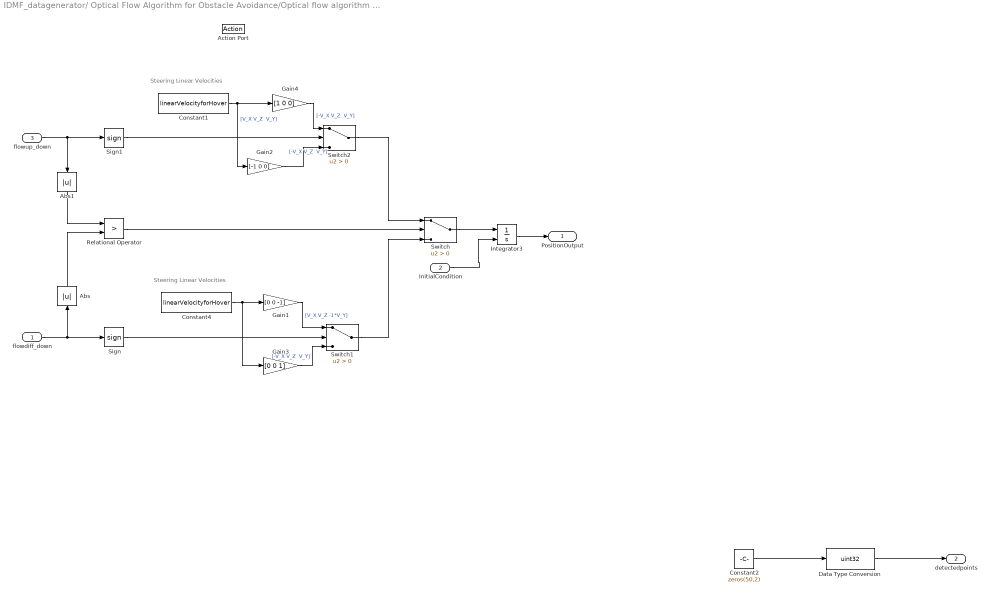
== system IDMF_datagenerator/ Optical Flow Algorithm for Obstacle Avoidance/Optical flow algorithm and PID Controller for landing/DronePositionEstimation.DroneHover ==
  note: Steering Linear Velocities
  note: Steering Linear Velocities
  flowdiff_down : Inport
  InitialCondition : Inport  Port=2
  flowup_down : Inport  Port=3
  Action Port : ActionPort
      settings: CopyFcn=Stateflow.SLINSF.SimulinkMan.removeBlockPreDeleteFcn  PreDeleteFcn=Stateflow.SLINSF.SimulinkMan.unsafePredeleteFcn
  Abs : Abs  SaturateOnIntegerOverflow=off
  Abs1 : Abs  SaturateOnIntegerOverflow=off
  Constant1 : Constant  Value=linearVelocityforHover
  Constant2 : Constant  Value=zeros(50,2)
  Constant4 : Constant  Value=linearVelocityforHover
  Data Type Conversion : DataTypeConversion  OutDataTypeStr=uint32  SaturateOnIntegerOverflow=off  RndMeth=Floor
  Gain1 : Gain  Gain=[0 0 -1]
  Gain2 : Gain  Gain=[-1 0 0]
  Gain3 : Gain  Gain=[0 0 1]
  Gain4 : Gain  Gain=[1 0 0]
  Integrator3 : Integrator  InitialConditionSource=external
  Relational Operator : RelationalOperator  Operator=>  OutDataTypeStr=boolean  RndMeth=Simplest  InputSameDT=off
  Sign : Signum
  Sign1 : Signum
  Switch : Switch  Criteria=u2 > Threshold  SaturateOnIntegerOverflow=off  InputSameDT=off
  Switch1 : Switch  Criteria=u2 > Threshold  SaturateOnIntegerOverflow=off  InputSameDT=off
  Switch2 : Switch  Criteria=u2 > Threshold  SaturateOnIntegerOverflow=off  InputSameDT=off
  PositionOutput : Outport
  detectedpoints : Outport  Port=2
      settings: VarSizeSig=Yes
  wires:
  Sign/1 -> Switch1/2
  Constant4/1 -> Gain3/1, Gain1/1
  Gain1/1 -> Switch1/1  "[V_X V_Z -1*V_Y]"
  flowdiff_down/1 -> Sign/1, Abs/1
  Integrator3/1 -> PositionOutput/1
  InitialCondition/1 -> Integrator3/2
  Sign1/1 -> Switch2/2
  Constant1/1 -> Gain4/1, Gain2/1  "[V_X V_Z  V_Y]"
  Switch2/1 -> Switch/1
  Abs/1 -> Relational Operator/2
  Abs1/1 -> Relational Operator/1
  Gain2/1 -> Switch2/3  "[-V_X V_Z  V_Y]"
  Switch/1 -> Integrator3/1
  Switch1/1 -> Switch/3
  Gain3/1 -> Switch1/3  "[-V_X V_Z  V_Y]"
  Gain4/1 -> Switch2/1  "[-V_X V_Z  V_Y]"
  Relational Operator/1 -> Switch/2
  flowup_down/1 -> Sign1/1, Abs1/1
  Constant2/1 -> Data Type Conversion/1
  Data Type Conversion/1 -> detectedpoints/1

== system IDMF_datagenerator/ Optical Flow Algorithm for Obstacle Avoidance/Optical flow algorithm and PID Controller for landing/DronePositionEstimation.DroneHover1 ==
  note: Eventually, after the X and Y locations have been reached, we decrease the height fron finalHoverHeight to the height of the helipad platform
  note: If the output from the Sign block is Positive, drone should move towards the left side, i.e. V_y is Negative. Also, if the output from the Sign block is Negative, drone will move towwars the right side..ie, V_y is Positive.
  note: Steering Linear Velocities
  flowdiff_down : Inport
  InitialCondition : Inport  Port=2
  Action Port : ActionPort
      settings: CopyFcn=Stateflow.SLINSF.SimulinkMan.removeBlockPreDeleteFcn  PreDeleteFcn=Stateflow.SLINSF.SimulinkMan.unsafePredeleteFcn
  Constant : Constant  Value=zeros(50,2)
  Constant4 : Constant  Value=linearVelocityforHover
  Data Type Conversion : DataTypeConversion  OutDataTypeStr=uint32  SaturateOnIntegerOverflow=off  RndMeth=Floor
  Gain1 : Gain  Gain=[1 0 -1]
  Gain3 : Gain  Gain=[1 0 1]
  Integrator3 : Integrator  InitialConditionSource=external
  Sign : Signum
  Switch1 : Switch  Criteria=u2 > Threshold  SaturateOnIntegerOverflow=off  InputSameDT=off
  PositionOutput : Outport
  detectedpoints : Outport  Port=2
      settings: VarSizeSig=Yes
  wires:
  Sign/1 -> Switch1/2
  Constant4/1 -> Gain3/1, Gain1/1
  Gain1/1 -> Switch1/1  "[V_X V_Z -1*V_Y]"
  flowdiff_down/1 -> Sign/1
  Integrator3/1 -> PositionOutput/1
  InitialCondition/1 -> Integrator3/2
  Switch1/1 -> Integrator3/1
  Gain3/1 -> Switch1/3  "[-V_X V_Z  V_Y]"
  Constant/1 -> Data Type Conversion/1
  Data Type Conversion/1 -> detectedpoints/1
